simulink model "NHTSA_LDW_Straight_dashed_left_cs"  (Simulink 7.6)
settings: Solver=ode5  SolverMode=SingleTasking  StartTime=0.0  StopTime=20  FixedStep=1/100  RelTol=1e-3
PreLoadFcn:
  | check_NUTS_defined;
  | 
  | assignin('base',['model_closed_' bdroot],false);
  | 
  | if exist('LDW_mask_sfun.mexw64')==3
  | delete LDW_mask_sfun.mexw64;
  | end
  | 
  | if exist('LDW_mask_sfun.mexw32') ==3
  | delete LDW_mask_sfun.mexw32;
  | end
  | 
  | switch version('-release')
  | case {'2010a', '2010b', '2011a'}
  | addpath('../includes_LKAS/includes_LKAS_2010a');
  | case {'2011b', '2012a', '2012b'}
  | addpath('../includes_LKAS/includes_LKAS_2011b');
  | otherwise
  | addpath('../includes_LKAS/includes_LKAS_2011b');
  | end
InitFcn:
  | PreScanExperimentInitFcn(bdroot)
StopFcn:
  | PreScanExperimentStopFcn(bdroot)
undefined symbols (not defined in the file): DiscIntNeverNeededParam, InitImageOutputDir, x_ini_VRML, y_ini_VRML, z_ini_VRML
libraries: simulink x22, PreScanSimulinkLibrary x8, simulink_extras x6, dspsnks4 x2, PreScanUsefulBlocks x2, simulink_need_slupdate x1
(part 3 of 5)

== system NHTSA_LDW_Straight_dashed_left_cs/VISULightSource_Audi_A8_1/conv_FogLightFrontRight ==
  on_off : Inport
  OffColor : Constant  Value="[51   51   51  255   77   77   77  255  102  102  102  255    0    0    0  255]"
  OnColor : Constant  Value="[51   51   51  255  204  204  204  255  102  102  102  255  510  510  510  255]"
  Switch1 : Switch  Threshold=0.5
  RGBcolor : Outport
  wires:
  OffColor/1 -> Switch1/3  "off"
  OnColor/1 -> Switch1/1  "on"
  on_off/1 -> Switch1/2
  Switch1/1 -> RGBcolor/1

== system NHTSA_LDW_Straight_dashed_left_cs/VISULightSource_Audi_A8_1/conv_FogLightRearLeft ==
  on_off : Inport
  OffColor : Constant  Value="[51   51   51  255   92    0    0  255  102  102  102  255    0    0    0  255]"
  OnColor : Constant  Value="[51   51   51  255  332   51    0  255  102  102  102  255  583   10    0  255]"
  Switch1 : Switch  Threshold=0.5
  RGBcolor : Outport
  wires:
  OffColor/1 -> Switch1/3  "off"
  OnColor/1 -> Switch1/1  "on"
  on_off/1 -> Switch1/2
  Switch1/1 -> RGBcolor/1

== system NHTSA_LDW_Straight_dashed_left_cs/VISULightSource_Audi_A8_1/conv_FogLightRearRight ==
  on_off : Inport
  OffColor : Constant  Value="[51   51   51  255   92    0    0  255  102  102  102  255    0    0    0  255]"
  OnColor : Constant  Value="[51   51   51  255  332   51    0  255  102  102  102  255  583   10    0  255]"
  Switch1 : Switch  Threshold=0.5
  RGBcolor : Outport
  wires:
  OffColor/1 -> Switch1/3  "off"
  OnColor/1 -> Switch1/1  "on"
  on_off/1 -> Switch1/2
  Switch1/1 -> RGBcolor/1

== system NHTSA_LDW_Straight_dashed_left_cs/VISULightSource_Audi_A8_1/conv_IndicatorLightsLeft ==
  on_off : Inport
  OffColor : Constant  Value="[51   51   51  255  138   69    0  255  102  102  102  255    0    0    0  255]"
  OnColor : Constant  Value="[51   51   51  255  255  128    0  255  102  102  102  255  255  191    0  255]"
  Switch1 : Switch  Threshold=0.5
  RGBcolor : Outport
  wires:
  Switch1/1 -> RGBcolor/1
  on_off/1 -> Switch1/2
  OnColor/1 -> Switch1/1  "on"
  OffColor/1 -> Switch1/3  "off"

== system NHTSA_LDW_Straight_dashed_left_cs/VISULightSource_Audi_A8_1/conv_IndicatorLightsRight ==
  on_off : Inport
  OffColor : Constant  Value="[51   51   51  255  138   69    0  255  102  102  102  255    0    0    0  255]"
  OnColor : Constant  Value="[51   51   51  255  255  128    0  255  102  102  102  255  255  191    0  255]"
  Switch1 : Switch  Threshold=0.5
  RGBcolor : Outport
  wires:
  OffColor/1 -> Switch1/3  "off"
  OnColor/1 -> Switch1/1  "on"
  on_off/1 -> Switch1/2
  Switch1/1 -> RGBcolor/1

== system NHTSA_LDW_Straight_dashed_left_cs/VISULightSource_Audi_A8_1/conv_MainLightFrontLeft ==
  on_off : Inport
  OffColor : Constant  Value="[26   26   26  255   77   77   77  255  102  102  102  255    0    0    0  255]"
  OnColor : Constant  Value="[51   51   51  255  255  255  255  255  102  102  102  255  683  683  683  255]"
  Switch1 : Switch  Threshold=0.5
  RGBcolor : Outport
  wires:
  OffColor/1 -> Switch1/3  "off"
  OnColor/1 -> Switch1/1  "on"
  on_off/1 -> Switch1/2
  Switch1/1 -> RGBcolor/1

== system NHTSA_LDW_Straight_dashed_left_cs/VISULightSource_Audi_A8_1/conv_MainLightFrontRight ==
  on_off : Inport
  OffColor : Constant  Value="[26   26   26  255   77   77   77  255  102  102  102  255    0    0    0  255]"
  OnColor : Constant  Value="[51   51   51  255  255  255  255  255  102  102  102  255  683  683  683  255]"
  Switch1 : Switch  Threshold=0.5
  RGBcolor : Outport
  wires:
  OffColor/1 -> Switch1/3  "off"
  OnColor/1 -> Switch1/1  "on"
  on_off/1 -> Switch1/2
  Switch1/1 -> RGBcolor/1

== system NHTSA_LDW_Straight_dashed_left_cs/VISULightSource_Audi_A8_1/conv_MainLightRearLeft ==
  on_off : Inport
  OffColor : Constant  Value="[51   51   51  255   92    0    0  255  102  102  102  255    0    0    0  255]"
  OnColor : Constant  Value="[51   51   51  255  322   51    0  255  102  102  102  255  255   40    0  255]"
  Switch1 : Switch  Threshold=0.5
  RGBcolor : Outport
  wires:
  OffColor/1 -> Switch1/3  "off"
  OnColor/1 -> Switch1/1  "on"
  on_off/1 -> Switch1/2
  Switch1/1 -> RGBcolor/1

== system NHTSA_LDW_Straight_dashed_left_cs/VISULightSource_Audi_A8_1/conv_MainLightRearRight ==
  on_off : Inport
  OffColor : Constant  Value="[51   51   51  255   92    0    0  255  102  102  102  255    0    0    0  255]"
  OnColor : Constant  Value="[51   51   51  255  322   51    0  255  102  102  102  255  255   40    0  255]"
  Switch1 : Switch  Threshold=0.5
  RGBcolor : Outport
  wires:
  OffColor/1 -> Switch1/3  "off"
  OnColor/1 -> Switch1/1  "on"
  on_off/1 -> Switch1/2
  Switch1/1 -> RGBcolor/1

== system NHTSA_LDW_Straight_dashed_left_cs/VISULightSource_Audi_A8_1/visu_BrakeLightLeft_0 ==
  Y : Inport
  Assignment : Assignment  IndexMode=Zero-based  SampleTime=TimeStep  IndexOptions=Starting index (dialog)  Indices=PortIndex  OutputSizes=[1 1]
  Data Store Read : DataStoreRead  DataStoreName=SimCoreActuators  SampleTime=TimeStep
  Data Store Write : DataStoreWrite  DataStoreName=SimCoreActuators
  wires:
  Y/1 -> Assignment/2
  Data Store Read/1 -> Assignment/1
  Assignment/1 -> Data Store Write/1

== system NHTSA_LDW_Straight_dashed_left_cs/VISULightSource_Audi_A8_1/visu_BrakeLightRight_0 ==
  Y : Inport
  Assignment : Assignment  IndexMode=Zero-based  SampleTime=TimeStep  IndexOptions=Starting index (dialog)  Indices=PortIndex  OutputSizes=[1 1]
  Data Store Read : DataStoreRead  DataStoreName=SimCoreActuators  SampleTime=TimeStep
  Data Store Write : DataStoreWrite  DataStoreName=SimCoreActuators
  wires:
  Y/1 -> Assignment/2
  Data Store Read/1 -> Assignment/1
  Assignment/1 -> Data Store Write/1

== system NHTSA_LDW_Straight_dashed_left_cs/VISULightSource_Audi_A8_1/visu_FogLightFrontLeft_0 ==
  Y : Inport
  Assignment : Assignment  IndexMode=Zero-based  SampleTime=TimeStep  IndexOptions=Starting index (dialog)  Indices=PortIndex  OutputSizes=[1 1]
  Data Store Read : DataStoreRead  DataStoreName=SimCoreActuators  SampleTime=TimeStep
  Data Store Write : DataStoreWrite  DataStoreName=SimCoreActuators
  wires:
  Y/1 -> Assignment/2
  Data Store Read/1 -> Assignment/1
  Assignment/1 -> Data Store Write/1

== system NHTSA_LDW_Straight_dashed_left_cs/VISULightSource_Audi_A8_1/visu_FogLightFrontRight_0 ==
  Y : Inport
  Assignment : Assignment  IndexMode=Zero-based  SampleTime=TimeStep  IndexOptions=Starting index (dialog)  Indices=PortIndex  OutputSizes=[1 1]
  Data Store Read : DataStoreRead  DataStoreName=SimCoreActuators  SampleTime=TimeStep
  Data Store Write : DataStoreWrite  DataStoreName=SimCoreActuators
  wires:
  Y/1 -> Assignment/2
  Data Store Read/1 -> Assignment/1
  Assignment/1 -> Data Store Write/1

== system NHTSA_LDW_Straight_dashed_left_cs/VISULightSource_Audi_A8_1/visu_FogLightRearLeft_0 ==
  Y : Inport
  Assignment : Assignment  IndexMode=Zero-based  SampleTime=TimeStep  IndexOptions=Starting index (dialog)  Indices=PortIndex  OutputSizes=[1 1]
  Data Store Read : DataStoreRead  DataStoreName=SimCoreActuators  SampleTime=TimeStep
  Data Store Write : DataStoreWrite  DataStoreName=SimCoreActuators
  wires:
  Y/1 -> Assignment/2
  Data Store Read/1 -> Assignment/1
  Assignment/1 -> Data Store Write/1

== system NHTSA_LDW_Straight_dashed_left_cs/VISULightSource_Audi_A8_1/visu_FogLightRearRight_0 ==
  Y : Inport
  Assignment : Assignment  IndexMode=Zero-based  SampleTime=TimeStep  IndexOptions=Starting index (dialog)  Indices=PortIndex  OutputSizes=[1 1]
  Data Store Read : DataStoreRead  DataStoreName=SimCoreActuators  SampleTime=TimeStep
  Data Store Write : DataStoreWrite  DataStoreName=SimCoreActuators
  wires:
  Y/1 -> Assignment/2
  Data Store Read/1 -> Assignment/1
  Assignment/1 -> Data Store Write/1

== system NHTSA_LDW_Straight_dashed_left_cs/VISULightSource_Audi_A8_1/visu_IndicatorLightsLeft_0 ==
  Y : Inport
  Assignment : Assignment  IndexMode=Zero-based  SampleTime=TimeStep  IndexOptions=Starting index (dialog)  Indices=PortIndex  OutputSizes=[1 1]
  Data Store Read : DataStoreRead  DataStoreName=SimCoreActuators  SampleTime=TimeStep
  Data Store Write : DataStoreWrite  DataStoreName=SimCoreActuators
  wires:
  Assignment/1 -> Data Store Write/1
  Data Store Read/1 -> Assignment/1
  Y/1 -> Assignment/2

== system NHTSA_LDW_Straight_dashed_left_cs/VISULightSource_Audi_A8_1/visu_IndicatorLightsRight_0 ==
  Y : Inport
  Assignment : Assignment  IndexMode=Zero-based  SampleTime=TimeStep  IndexOptions=Starting index (dialog)  Indices=PortIndex  OutputSizes=[1 1]
  Data Store Read : DataStoreRead  DataStoreName=SimCoreActuators  SampleTime=TimeStep
  Data Store Write : DataStoreWrite  DataStoreName=SimCoreActuators
  wires:
  Y/1 -> Assignment/2
  Data Store Read/1 -> Assignment/1
  Assignment/1 -> Data Store Write/1

== system NHTSA_LDW_Straight_dashed_left_cs/VISULightSource_Audi_A8_1/visu_MainLightFrontLeft_0 ==
  Y : Inport
  Assignment : Assignment  IndexMode=Zero-based  SampleTime=TimeStep  IndexOptions=Starting index (dialog)  Indices=PortIndex  OutputSizes=[1 1]
  Data Store Read : DataStoreRead  DataStoreName=SimCoreActuators  SampleTime=TimeStep
  Data Store Write : DataStoreWrite  DataStoreName=SimCoreActuators
  wires:
  Y/1 -> Assignment/2
  Data Store Read/1 -> Assignment/1
  Assignment/1 -> Data Store Write/1

== system NHTSA_LDW_Straight_dashed_left_cs/VISULightSource_Audi_A8_1/visu_MainLightFrontRight_0 ==
  Y : Inport
  Assignment : Assignment  IndexMode=Zero-based  SampleTime=TimeStep  IndexOptions=Starting index (dialog)  Indices=PortIndex  OutputSizes=[1 1]
  Data Store Read : DataStoreRead  DataStoreName=SimCoreActuators  SampleTime=TimeStep
  Data Store Write : DataStoreWrite  DataStoreName=SimCoreActuators
  wires:
  Y/1 -> Assignment/2
  Data Store Read/1 -> Assignment/1
  Assignment/1 -> Data Store Write/1

== system NHTSA_LDW_Straight_dashed_left_cs/VISULightSource_Audi_A8_1/visu_MainLightRearLeft_0 ==
  Y : Inport
  Assignment : Assignment  IndexMode=Zero-based  SampleTime=TimeStep  IndexOptions=Starting index (dialog)  Indices=PortIndex  OutputSizes=[1 1]
  Data Store Read : DataStoreRead  DataStoreName=SimCoreActuators  SampleTime=TimeStep
  Data Store Write : DataStoreWrite  DataStoreName=SimCoreActuators
  wires:
  Y/1 -> Assignment/2
  Data Store Read/1 -> Assignment/1
  Assignment/1 -> Data Store Write/1

== system NHTSA_LDW_Straight_dashed_left_cs/VISULightSource_Audi_A8_1/visu_MainLightRearRight_0 ==
  Y : Inport
  Assignment : Assignment  IndexMode=Zero-based  SampleTime=TimeStep  IndexOptions=Starting index (dialog)  Indices=PortIndex  OutputSizes=[1 1]
  Data Store Read : DataStoreRead  DataStoreName=SimCoreActuators  SampleTime=TimeStep
  Data Store Write : DataStoreWrite  DataStoreName=SimCoreActuators
  wires:
  Y/1 -> Assignment/2
  Data Store Read/1 -> Assignment/1
  Assignment/1 -> Data Store Write/1

== system NHTSA_LDW_Straight_dashed_left_cs/VISUSteer_Audi_A8_1/conv_SteeringColumn ==
  angle [deg] : Inport
  Constant13 : Constant  Value=[0 1 0]
  Mux8 : Mux  Inputs=2
  deg2rad : Gain  Gain=pi/180
  QuaternionVisu [rad] : Outport
  wires:
  deg2rad/1 -> Mux8/2
  Constant13/1 -> Mux8/1
  Mux8/1 -> QuaternionVisu [rad]/1
  angle [deg]/1 -> deg2rad/1

== system NHTSA_LDW_Straight_dashed_left_cs/VISUSteer_Audi_A8_1/conv_SteeringWheel ==
  angle [deg] : Inport
  Constant13 : Constant  Value=[-1 0 0]
  Mux8 : Mux  Inputs=2
  deg2rad : Gain  Gain=pi/180
  QuaternionVisu [rad] : Outport
  wires:
  deg2rad/1 -> Mux8/2
  Constant13/1 -> Mux8/1
  Mux8/1 -> QuaternionVisu [rad]/1
  angle [deg]/1 -> deg2rad/1

== system NHTSA_LDW_Straight_dashed_left_cs/VISUSteer_Audi_A8_1/visu_SteeringColumn ==
  Y : Inport
  Assignment : Assignment  IndexMode=Zero-based  SampleTime=TimeStep  IndexOptions=Starting index (dialog)  Indices=PortIndex  OutputSizes=[1 1]
  Data Store Read : DataStoreRead  DataStoreName=SimCoreActuators  SampleTime=TimeStep
  Data Store Write : DataStoreWrite  DataStoreName=SimCoreActuators
  wires:
  Assignment/1 -> Data Store Write/1
  Data Store Read/1 -> Assignment/1
  Y/1 -> Assignment/2

== system NHTSA_LDW_Straight_dashed_left_cs/VISUSteer_Audi_A8_1/visu_SteeringWheel ==
  Y : Inport
  Assignment : Assignment  IndexMode=Zero-based  SampleTime=TimeStep  IndexOptions=Starting index (dialog)  Indices=PortIndex  OutputSizes=[1 1]
  Data Store Read : DataStoreRead  DataStoreName=SimCoreActuators  SampleTime=TimeStep
  Data Store Write : DataStoreWrite  DataStoreName=SimCoreActuators
  wires:
  Assignment/1 -> Data Store Write/1
  Data Store Read/1 -> Assignment/1
  Y/1 -> Assignment/2

== system NHTSA_LDW_Straight_dashed_left_cs/VISUWheels_Audi_A8_1/conv_RotWheelFL ==
  BryantISO [deg] : Inport
  Fcn10 : Fcn  Expr=cos(u(1))*sin(u(3))+sin(u(1))*sin(u(2))*cos(u(3))
  Fcn11 : Fcn  Expr=sin(u(1))*sin(u(3))-cos(u(1))*sin(u(2))*cos(u(3))
  Fcn12 : Fcn  Expr=-cos(u(2))*sin(u(3))
  Fcn13 : Fcn  Expr=cos(u(1))*cos(u(3))-sin(u(1))*sin(u(2))*sin(u(3))
  Fcn14 : Fcn  Expr=sin(u(1))*cos(u(3))+cos(u(1))*sin(u(2))*sin(u(3))
  Fcn15 : Fcn  Expr=sin(u(2))
  Fcn16 : Fcn  Expr=-sin(u(1))*cos(u(2))
  Fcn17 : Fcn  Expr=cos(u(1))*cos(u(2))
  Fcn9 : Fcn  Expr=cos(u(2))*cos(u(3))
  Mux1 : Mux  Inputs=9
  RotMat2AxisAngle : Subsystem
  deg2rad : Gain  Gain=pi/180
  xyz 2 zxy : Selector  InputPortWidth=3  IndexOptions=Index vector (dialog)  Indices=[3 1 2]  OutputSizes=1
  zxy 2 xyz : Selector  InputPortWidth=4  IndexOptions=Index vector (dialog)  Indices=[2 3 1 4]  OutputSizes=1
  QuaternionVisu [rad] : Outport
  wires:
  zxy 2 xyz/1 -> QuaternionVisu [rad]/1
  xyz 2 zxy/1 -> deg2rad/1
  deg2rad/1 -> Fcn17/1, Fcn16/1, Fcn15/1, Fcn14/1, Fcn13/1, Fcn12/1, Fcn11/1, Fcn10/1, Fcn9/1
  BryantISO [deg]/1 -> xyz 2 zxy/1  "BryantAngles rotx roty rotz Visu"
  RotMat2AxisAngle/1(Angles_Visu) -> zxy 2 xyz/1
  Mux1/1 -> RotMat2AxisAngle/1(RotMat_Visu)  "RotationMatrix Visu"
  Fcn17/1 -> Mux1/9
  Fcn16/1 -> Mux1/8
  Fcn15/1 -> Mux1/7
  Fcn14/1 -> Mux1/6
  Fcn13/1 -> Mux1/5
  Fcn12/1 -> Mux1/4
  Fcn11/1 -> Mux1/3
  Fcn10/1 -> Mux1/2
  Fcn9/1 -> Mux1/1

== system NHTSA_LDW_Straight_dashed_left_cs/VISUWheels_Audi_A8_1/conv_RotWheelFR ==
  BryantISO [deg] : Inport
  Fcn10 : Fcn  Expr=cos(u(1))*sin(u(3))+sin(u(1))*sin(u(2))*cos(u(3))
  Fcn11 : Fcn  Expr=sin(u(1))*sin(u(3))-cos(u(1))*sin(u(2))*cos(u(3))
  Fcn12 : Fcn  Expr=-cos(u(2))*sin(u(3))
  Fcn13 : Fcn  Expr=cos(u(1))*cos(u(3))-sin(u(1))*sin(u(2))*sin(u(3))
  Fcn14 : Fcn  Expr=sin(u(1))*cos(u(3))+cos(u(1))*sin(u(2))*sin(u(3))
  Fcn15 : Fcn  Expr=sin(u(2))
  Fcn16 : Fcn  Expr=-sin(u(1))*cos(u(2))
  Fcn17 : Fcn  Expr=cos(u(1))*cos(u(2))
  Fcn9 : Fcn  Expr=cos(u(2))*cos(u(3))
  Mux1 : Mux  Inputs=9
  RotMat2AxisAngle : Subsystem
  deg2rad : Gain  Gain=pi/180
  xyz 2 zxy : Selector  InputPortWidth=3  IndexOptions=Index vector (dialog)  Indices=[3 1 2]  OutputSizes=1
  zxy 2 xyz : Selector  InputPortWidth=4  IndexOptions=Index vector (dialog)  Indices=[2 3 1 4]  OutputSizes=1
  QuaternionVisu [rad] : Outport
  wires:
  zxy 2 xyz/1 -> QuaternionVisu [rad]/1
  xyz 2 zxy/1 -> deg2rad/1
  deg2rad/1 -> Fcn17/1, Fcn16/1, Fcn15/1, Fcn14/1, Fcn13/1, Fcn12/1, Fcn11/1, Fcn10/1, Fcn9/1
  BryantISO [deg]/1 -> xyz 2 zxy/1  "BryantAngles rotx roty rotz Visu"
  RotMat2AxisAngle/1(Angles_Visu) -> zxy 2 xyz/1
  Mux1/1 -> RotMat2AxisAngle/1(RotMat_Visu)  "RotationMatrix Visu"
  Fcn17/1 -> Mux1/9
  Fcn16/1 -> Mux1/8
  Fcn15/1 -> Mux1/7
  Fcn14/1 -> Mux1/6
  Fcn13/1 -> Mux1/5
  Fcn12/1 -> Mux1/4
  Fcn11/1 -> Mux1/3
  Fcn10/1 -> Mux1/2
  Fcn9/1 -> Mux1/1

== system NHTSA_LDW_Straight_dashed_left_cs/VISUWheels_Audi_A8_1/conv_RotWheelRL ==
  BryantISO [deg] : Inport
  Fcn10 : Fcn  Expr=cos(u(1))*sin(u(3))+sin(u(1))*sin(u(2))*cos(u(3))
  Fcn11 : Fcn  Expr=sin(u(1))*sin(u(3))-cos(u(1))*sin(u(2))*cos(u(3))
  Fcn12 : Fcn  Expr=-cos(u(2))*sin(u(3))
  Fcn13 : Fcn  Expr=cos(u(1))*cos(u(3))-sin(u(1))*sin(u(2))*sin(u(3))
  Fcn14 : Fcn  Expr=sin(u(1))*cos(u(3))+cos(u(1))*sin(u(2))*sin(u(3))
  Fcn15 : Fcn  Expr=sin(u(2))
  Fcn16 : Fcn  Expr=-sin(u(1))*cos(u(2))
  Fcn17 : Fcn  Expr=cos(u(1))*cos(u(2))
  Fcn9 : Fcn  Expr=cos(u(2))*cos(u(3))
  Mux1 : Mux  Inputs=9
  RotMat2AxisAngle : Subsystem
  deg2rad : Gain  Gain=pi/180
  xyz 2 zxy : Selector  InputPortWidth=3  IndexOptions=Index vector (dialog)  Indices=[3 1 2]  OutputSizes=1
  zxy 2 xyz : Selector  InputPortWidth=4  IndexOptions=Index vector (dialog)  Indices=[2 3 1 4]  OutputSizes=1
  QuaternionVisu [rad] : Outport
  wires:
  zxy 2 xyz/1 -> QuaternionVisu [rad]/1
  xyz 2 zxy/1 -> deg2rad/1
  deg2rad/1 -> Fcn17/1, Fcn16/1, Fcn15/1, Fcn14/1, Fcn13/1, Fcn12/1, Fcn11/1, Fcn10/1, Fcn9/1
  BryantISO [deg]/1 -> xyz 2 zxy/1  "BryantAngles rotx roty rotz Visu"
  RotMat2AxisAngle/1(Angles_Visu) -> zxy 2 xyz/1
  Mux1/1 -> RotMat2AxisAngle/1(RotMat_Visu)  "RotationMatrix Visu"
  Fcn17/1 -> Mux1/9
  Fcn16/1 -> Mux1/8
  Fcn15/1 -> Mux1/7
  Fcn14/1 -> Mux1/6
  Fcn13/1 -> Mux1/5
  Fcn12/1 -> Mux1/4
  Fcn11/1 -> Mux1/3
  Fcn10/1 -> Mux1/2
  Fcn9/1 -> Mux1/1

== system NHTSA_LDW_Straight_dashed_left_cs/VISUWheels_Audi_A8_1/conv_RotWheelRR ==
  BryantISO [deg] : Inport
  Fcn10 : Fcn  Expr=cos(u(1))*sin(u(3))+sin(u(1))*sin(u(2))*cos(u(3))
  Fcn11 : Fcn  Expr=sin(u(1))*sin(u(3))-cos(u(1))*sin(u(2))*cos(u(3))
  Fcn12 : Fcn  Expr=-cos(u(2))*sin(u(3))
  Fcn13 : Fcn  Expr=cos(u(1))*cos(u(3))-sin(u(1))*sin(u(2))*sin(u(3))
  Fcn14 : Fcn  Expr=sin(u(1))*cos(u(3))+cos(u(1))*sin(u(2))*sin(u(3))
  Fcn15 : Fcn  Expr=sin(u(2))
  Fcn16 : Fcn  Expr=-sin(u(1))*cos(u(2))
  Fcn17 : Fcn  Expr=cos(u(1))*cos(u(2))
  Fcn9 : Fcn  Expr=cos(u(2))*cos(u(3))
  Mux1 : Mux  Inputs=9
  RotMat2AxisAngle : Subsystem
  deg2rad : Gain  Gain=pi/180
  xyz 2 zxy : Selector  InputPortWidth=3  IndexOptions=Index vector (dialog)  Indices=[3 1 2]  OutputSizes=1
  zxy 2 xyz : Selector  InputPortWidth=4  IndexOptions=Index vector (dialog)  Indices=[2 3 1 4]  OutputSizes=1
  QuaternionVisu [rad] : Outport
  wires:
  zxy 2 xyz/1 -> QuaternionVisu [rad]/1
  xyz 2 zxy/1 -> deg2rad/1
  deg2rad/1 -> Fcn17/1, Fcn16/1, Fcn15/1, Fcn14/1, Fcn13/1, Fcn12/1, Fcn11/1, Fcn10/1, Fcn9/1
  BryantISO [deg]/1 -> xyz 2 zxy/1  "BryantAngles rotx roty rotz Visu"
  RotMat2AxisAngle/1(Angles_Visu) -> zxy 2 xyz/1
  Mux1/1 -> RotMat2AxisAngle/1(RotMat_Visu)  "RotationMatrix Visu"
  Fcn17/1 -> Mux1/9
  Fcn16/1 -> Mux1/8
  Fcn15/1 -> Mux1/7
  Fcn14/1 -> Mux1/6
  Fcn13/1 -> Mux1/5
  Fcn12/1 -> Mux1/4
  Fcn11/1 -> Mux1/3
  Fcn10/1 -> Mux1/2
  Fcn9/1 -> Mux1/1

== system NHTSA_LDW_Straight_dashed_left_cs/VISUWheels_Audi_A8_1/conv_TransWheelFL ==
  transISO [m] : Inport
  Gain1 : Gain  Gain=Gain_xISO
  Gain2 : Gain  Gain=Gain_yISO
  Gain3 : Gain  Gain=Gain_zISO
  Mux2 : Mux  Inputs=3
  Sum : Sum  Inputs=|++
  pos_ini_Visu : Subsystem
  transISO2Visu : Subsystem
  transVisu [m] : Outport
  wires:
  Gain3/1 -> Mux2/3
  Gain2/1 -> Mux2/2
  Gain1/1 -> Mux2/1
  Sum/1 -> transVisu [m]/1
  pos_ini_Visu/1(pos_ini_Visu) -> Sum/2
  Mux2/1 -> Sum/1
  transISO [m]/1 -> transISO2Visu/1(transISO)
  transISO2Visu/1(trans_x_Visu) -> Gain1/1
  transISO2Visu/2(trans_y_Visu) -> Gain2/1
  transISO2Visu/3(trans_z_Visu) -> Gain3/1

== system NHTSA_LDW_Straight_dashed_left_cs/VISUWheels_Audi_A8_1/conv_TransWheelFR ==
  transISO [m] : Inport
  Gain1 : Gain  Gain=Gain_xISO
  Gain2 : Gain  Gain=Gain_yISO
  Gain3 : Gain  Gain=Gain_zISO
  Mux2 : Mux  Inputs=3
  Sum : Sum  Inputs=|++
  pos_ini_Visu : Subsystem
  transISO2Visu : Subsystem
  transVisu [m] : Outport
  wires:
  Gain3/1 -> Mux2/3
  Gain2/1 -> Mux2/2
  Gain1/1 -> Mux2/1
  Sum/1 -> transVisu [m]/1
  pos_ini_Visu/1(pos_ini_Visu) -> Sum/2
  Mux2/1 -> Sum/1
  transISO [m]/1 -> transISO2Visu/1(transISO)
  transISO2Visu/1(trans_x_Visu) -> Gain1/1
  transISO2Visu/2(trans_y_Visu) -> Gain2/1
  transISO2Visu/3(trans_z_Visu) -> Gain3/1

== system NHTSA_LDW_Straight_dashed_left_cs/VISUWheels_Audi_A8_1/conv_TransWheelRL ==
  transISO [m] : Inport
  Gain1 : Gain  Gain=Gain_xISO
  Gain2 : Gain  Gain=Gain_yISO
  Gain3 : Gain  Gain=Gain_zISO
  Mux2 : Mux  Inputs=3
  Sum : Sum  Inputs=|++
  pos_ini_Visu : Subsystem
  transISO2Visu : Subsystem
  transVisu [m] : Outport
  wires:
  Gain3/1 -> Mux2/3
  Gain2/1 -> Mux2/2
  Gain1/1 -> Mux2/1
  Sum/1 -> transVisu [m]/1
  pos_ini_Visu/1(pos_ini_Visu) -> Sum/2
  Mux2/1 -> Sum/1
  transISO2Visu/3(trans_z_Visu) -> Gain3/1
  transISO2Visu/2(trans_y_Visu) -> Gain2/1
  transISO [m]/1 -> transISO2Visu/1(transISO)
  transISO2Visu/1(trans_x_Visu) -> Gain1/1

== system NHTSA_LDW_Straight_dashed_left_cs/VISUWheels_Audi_A8_1/conv_TransWheelRR ==
  transISO [m] : Inport
  Gain1 : Gain  Gain=Gain_xISO
  Gain2 : Gain  Gain=Gain_yISO
  Gain3 : Gain  Gain=Gain_zISO
  Mux2 : Mux  Inputs=3
  Sum : Sum  Inputs=|++
  pos_ini_Visu : Subsystem
  transISO2Visu : Subsystem
  transVisu [m] : Outport
  wires:
  Gain3/1 -> Mux2/3
  Gain2/1 -> Mux2/2
  Gain1/1 -> Mux2/1
  Sum/1 -> transVisu [m]/1
  pos_ini_Visu/1(pos_ini_Visu) -> Sum/2
  Mux2/1 -> Sum/1
  transISO2Visu/3(trans_z_Visu) -> Gain3/1
  transISO2Visu/2(trans_y_Visu) -> Gain2/1
  transISO [m]/1 -> transISO2Visu/1(transISO)
  transISO2Visu/1(trans_x_Visu) -> Gain1/1

== system NHTSA_LDW_Straight_dashed_left_cs/VISUWheels_Audi_A8_1/visu_RotWheelFL ==
  Y : Inport
  Assignment : Assignment  IndexMode=Zero-based  SampleTime=TimeStep  IndexOptions=Starting index (dialog)  Indices=PortIndex  OutputSizes=[1 1]
  Data Store Read : DataStoreRead  DataStoreName=SimCoreActuators  SampleTime=TimeStep
  Data Store Write : DataStoreWrite  DataStoreName=SimCoreActuators
  wires:
  Y/1 -> Assignment/2
  Data Store Read/1 -> Assignment/1
  Assignment/1 -> Data Store Write/1

== system NHTSA_LDW_Straight_dashed_left_cs/VISUWheels_Audi_A8_1/visu_RotWheelFR ==
  Y : Inport
  Assignment : Assignment  IndexMode=Zero-based  SampleTime=TimeStep  IndexOptions=Starting index (dialog)  Indices=PortIndex  OutputSizes=[1 1]
  Data Store Read : DataStoreRead  DataStoreName=SimCoreActuators  SampleTime=TimeStep
  Data Store Write : DataStoreWrite  DataStoreName=SimCoreActuators
  wires:
  Y/1 -> Assignment/2
  Data Store Read/1 -> Assignment/1
  Assignment/1 -> Data Store Write/1

== system NHTSA_LDW_Straight_dashed_left_cs/VISUWheels_Audi_A8_1/visu_RotWheelRL ==
  Y : Inport
  Assignment : Assignment  IndexMode=Zero-based  SampleTime=TimeStep  IndexOptions=Starting index (dialog)  Indices=PortIndex  OutputSizes=[1 1]
  Data Store Read : DataStoreRead  DataStoreName=SimCoreActuators  SampleTime=TimeStep
  Data Store Write : DataStoreWrite  DataStoreName=SimCoreActuators
  wires:
  Y/1 -> Assignment/2
  Data Store Read/1 -> Assignment/1
  Assignment/1 -> Data Store Write/1

== system NHTSA_LDW_Straight_dashed_left_cs/VISUWheels_Audi_A8_1/visu_RotWheelRR ==
  Y : Inport
  Assignment : Assignment  IndexMode=Zero-based  SampleTime=TimeStep  IndexOptions=Starting index (dialog)  Indices=PortIndex  OutputSizes=[1 1]
  Data Store Read : DataStoreRead  DataStoreName=SimCoreActuators  SampleTime=TimeStep
  Data Store Write : DataStoreWrite  DataStoreName=SimCoreActuators
  wires:
  Y/1 -> Assignment/2
  Data Store Read/1 -> Assignment/1
  Assignment/1 -> Data Store Write/1

== system NHTSA_LDW_Straight_dashed_left_cs/VISUWheels_Audi_A8_1/visu_TransWheelFL ==
  Y : Inport
  Assignment : Assignment  IndexMode=Zero-based  SampleTime=TimeStep  IndexOptions=Starting index (dialog)  Indices=PortIndex  OutputSizes=[1 1]
  Data Store Read : DataStoreRead  DataStoreName=SimCoreActuators  SampleTime=TimeStep
  Data Store Write : DataStoreWrite  DataStoreName=SimCoreActuators
  wires:
  Y/1 -> Assignment/2
  Data Store Read/1 -> Assignment/1
  Assignment/1 -> Data Store Write/1

== system NHTSA_LDW_Straight_dashed_left_cs/VISUWheels_Audi_A8_1/visu_TransWheelFR ==
  Y : Inport
  Assignment : Assignment  IndexMode=Zero-based  SampleTime=TimeStep  IndexOptions=Starting index (dialog)  Indices=PortIndex  OutputSizes=[1 1]
  Data Store Read : DataStoreRead  DataStoreName=SimCoreActuators  SampleTime=TimeStep
  Data Store Write : DataStoreWrite  DataStoreName=SimCoreActuators
  wires:
  Y/1 -> Assignment/2
  Data Store Read/1 -> Assignment/1
  Assignment/1 -> Data Store Write/1

== system NHTSA_LDW_Straight_dashed_left_cs/VISUWheels_Audi_A8_1/visu_TransWheelRL ==
  Y : Inport
  Assignment : Assignment  IndexMode=Zero-based  SampleTime=TimeStep  IndexOptions=Starting index (dialog)  Indices=PortIndex  OutputSizes=[1 1]
  Data Store Read : DataStoreRead  DataStoreName=SimCoreActuators  SampleTime=TimeStep
  Data Store Write : DataStoreWrite  DataStoreName=SimCoreActuators
  wires:
  Y/1 -> Assignment/2
  Data Store Read/1 -> Assignment/1
  Assignment/1 -> Data Store Write/1

== system NHTSA_LDW_Straight_dashed_left_cs/VISUWheels_Audi_A8_1/visu_TransWheelRR ==
  Y : Inport
  Assignment : Assignment  IndexMode=Zero-based  SampleTime=TimeStep  IndexOptions=Starting index (dialog)  Indices=PortIndex  OutputSizes=[1 1]
  Data Store Read : DataStoreRead  DataStoreName=SimCoreActuators  SampleTime=TimeStep
  Data Store Write : DataStoreWrite  DataStoreName=SimCoreActuators
  wires:
  Y/1 -> Assignment/2
  Data Store Read/1 -> Assignment/1
  Assignment/1 -> Data Store Write/1

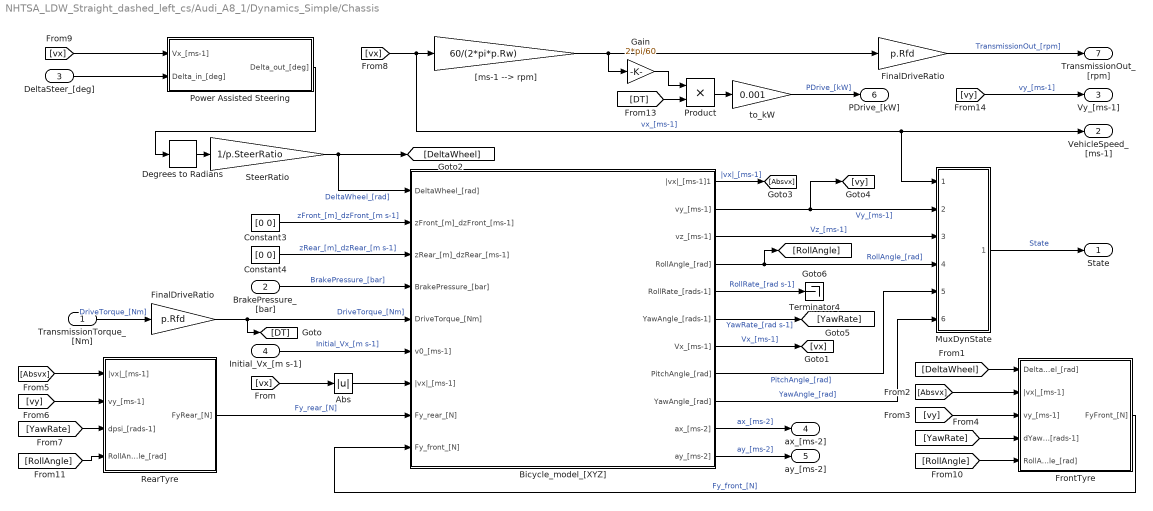
== system NHTSA_LDW_Straight_dashed_left_cs/Audi_A8_1/Dynamics_Simple/Chassis ==
  TransmissionTorque_[Nm] : Inport
  BrakePressure_[bar] : Inport  Port=2
  DeltaSteer_[deg] : Inport  Port=3
  Initial_Vx_[m s-1] : Inport  Port=4
  Abs : Abs
  Bicycle_model_[XYZ] : Subsystem
      mask Display: image(imread('Bicycle_model.png'));
  Constant3 : Constant  Value=[0 0]
  Constant4 : Constant  Value=[0 0]
  Degrees to Radians : simulink_extras/Transformations/Degrees to Radians  SystemSampleTime=-1
  FinalDriveRatio : Gain  Gain=p.Rfd  SaturateOnIntegerOverflow=on  OutDataTypeStr=Inherit: Same as input  ParamDataTypeStr=Inherit: Same as input
  "FinalDriveRatio " : Gain  Gain=p.Rfd  SaturateOnIntegerOverflow=on  OutDataTypeStr=Inherit: Same as input  ParamDataTypeStr=Inherit: Same as input
  FrontTyre : Subsystem
      mask Display: image(imread('Tyre.png'));
  Gain : Gain  Gain=2*pi/60
  MuxDynState : Subsystem
  Power Assisted Steering : Subsystem
  Product : Product  RndMeth=Zero
  RearTyre : Subsystem
      mask Display: image(imread('Tyre.png'));
  SteerRatio : Gain  Gain=1/p.SteerRatio
  Terminator4 : Terminator
  "[ms-1 --> rpm]" : Gain  Gain=60/(2*pi*p.Rw)  SaturateOnIntegerOverflow=on  OutDataTypeStr=Inherit: Same as input  ParamDataTypeStr=Inherit: Same as input
  to_kW : Gain  Gain=0.001
  State : Outport
  VehicleSpeed_[ms-1] : Outport  Port=2
  Vy_[ms-1] : Outport  Port=3
  ax_[ms-2] : Outport  Port=4
  ay_[ms-2] : Outport  Port=5
  PDrive_[kW] : Outport  Port=6
  TransmissionOut_[rpm] : Outport  Port=7
  wires:
  [vy] -> Vy_[ms-1]/1  "vy_[ms-1]"
  to_kW/1 -> PDrive_[kW]/1  "PDrive_[kW]"
  Gain/1 -> Product/1
  Bicycle_model_[XYZ]/10(ax_[ms-2]) -> ax_[ms-2]/1  "ax_[ms-2]"
  Product/1 -> to_kW/1
  [DT] -> Product/2
  Bicycle_model_[XYZ]/11(ay_[ms-2]) -> ay_[ms-2]/1  "ay_[ms-2]"
  Abs/1 -> Bicycle_model_[XYZ]/7(|vx|_[ms-1])
  Degrees to Radians/1 -> SteerRatio/1
  [vx] -> Abs/1
  SteerRatio/1 -> [DeltaWheel], Bicycle_model_[XYZ]/1(DeltaWheel_[rad])  "DeltaWheel_[rad]"
  TransmissionTorque_[Nm]/1 -> "FinalDriveRatio "/1  "DriveTorque_[Nm]"
  RearTyre/1(FyRear_[N]) -> Bicycle_model_[XYZ]/8(Fy_rear_[N])  "Fy_rear_[N]"
  FrontTyre/1(FyFront_[N]) -> Bicycle_model_[XYZ]/9(Fy_front_[N])  "Fy_front_[N]"
  Bicycle_model_[XYZ]/1(|vx|_[ms-1]1) -> [Absvx]  "|vx|_[ms-1]"
  Bicycle_model_[XYZ]/2(vy_[ms-1]) -> [vy], MuxDynState/2(vy [ms-1])  "Vy_[ms-1]"
  Bicycle_model_[XYZ]/4(RollAngle_[rad]) -> MuxDynState/4(R [rad]), [RollAngle]  "RollAngle_[rad]"
  Bicycle_model_[XYZ]/6(YawAngle_[rads-1]) -> [YawRate]  "YawRate_[rad s-1]"
  Bicycle_model_[XYZ]/7(Vx_[ms-1]) -> [vx]  "Vx_[ms-1]"
  [DeltaWheel] -> FrontTyre/1(DeltaWheel_[rad])
  [Absvx] -> FrontTyre/2(|vx|_[ms-1])
  [vy] -> FrontTyre/3(vy_[ms-1])
  [YawRate] -> FrontTyre/4(dYawAngle_[rads-1])
  [Absvx] -> RearTyre/1(|vx|_[ms-1])
  [vy] -> RearTyre/2(vy_[ms-1])
  [YawRate] -> RearTyre/3(dpsi_[rads-1])
  Bicycle_model_[XYZ]/3(vz_[ms-1]) -> MuxDynState/3(vz [ms-1])  "Vz_[ms-1]"
  Bicycle_model_[XYZ]/8(PitchAngle_[rad]) -> MuxDynState/5(P [rad])  "PitchAngle_[rad]"
  Bicycle_model_[XYZ]/9(YawAngle_[rad]) -> MuxDynState/6(Y [rad])  "YawAngle_[rad]"
  "[ms-1 --> rpm]"/1 -> Gain/1, FinalDriveRatio/1
  FinalDriveRatio/1 -> TransmissionOut_[rpm]/1  "TransmissionOut_[rpm]"
  [vx] -> "[ms-1 --> rpm]"/1, VehicleSpeed_[ms-1]/1, MuxDynState/1(vx [ms-1])  "vx_[ms-1]"
  [vx] -> Power Assisted Steering/1(Vx_[ms-1])
  DeltaSteer_[deg]/1 -> Power Assisted Steering/2(Delta_in_[deg])
  Power Assisted Steering/1(Delta_out_[deg]) -> Degrees to Radians/1
  [RollAngle] -> FrontTyre/5(RollAngle_[rad])
  [RollAngle] -> RearTyre/4(RollAngle_[rad])
  Constant3/1 -> Bicycle_model_[XYZ]/2(zFront_[m]_dzFront_[ms-1])  "zFront_[m]_dzFront_[m s-1]"
  Constant4/1 -> Bicycle_model_[XYZ]/3(zRear_[m]_dzRear_[ms-1])  "zRear_[m]_dzRear_[m s-1]"
  BrakePressure_[bar]/1 -> Bicycle_model_[XYZ]/4(BrakePressure_[bar])  "BrakePressure_[bar]"
  "FinalDriveRatio "/1 -> Bicycle_model_[XYZ]/5(DriveTorque_[Nm]), [DT]  "DriveTorque_[Nm]"
  Initial_Vx_[m s-1]/1 -> Bicycle_model_[XYZ]/6(v0_[ms-1])  "Initial_Vx_[m s-1]"
  Bicycle_model_[XYZ]/5(RollRate_[rads-1]) -> Terminator4/1  "RollRate_[rad s-1]"
  MuxDynState/1(State) -> State/1  "State"

== system NHTSA_LDW_Straight_dashed_left_cs/Audi_A8_1/Dynamics_Simple/Engine ==
  ImpellerTorque_[Nm] : Inport
  Throttle_[%] : Inport  Port=2
  Configurable Subsystem : Subsystem  BlockChoice=Discrete Rate Limiter  mask{ComputationMode=ComputationMode}
      mask prompts: ComputationMode "Compuation mode:"
      mask init:
      | SetComputationMode(gcb,ComputationMode);
      settings: AttributesFormatString=%<BlockChoice>  OpenFcn=BringToFront(gcb);  MemberBlocks=Discrete Rate Limiter,Rate Limiter
      settings: TemplateBlock=|
      | PreScanSimulinkLibrary/Configurable Subsystems/TransferFunction
      | Engine/Configurable
      | Subsystem
  Configurable Subsystem1 : Subsystem  BlockChoice=Discrete-Time Integrator  mask{ComputationMode=ComputationMode}
      mask prompts: ComputationMode "Computation mode:"
      mask init:
      | SetComputationMode(gcb,ComputationMode);
      settings: AttributesFormatString=%<BlockChoice>  OpenFcn=BringToFront(gcb);  MemberBlocks=Discrete-Time Integrator,Integrator
      settings: TemplateBlock=|
      | PreScanSimulinkLibrary/Configurable Subsystems/integral with initial condition and limts
      | for engine/Configurable
      | Subsystem
  EngineTorque : Lookup2D  RowIndex=p.thvec  ColumnIndex=p.nevec  Table=p.emap  InputSameDT=on
  Gain : Gain  Gain=2*pi/60
  Product : Product  RndMeth=Zero
  Sum : Sum  Inputs=-+  SaturateOnIntegerOverflow=on  InputSameDT=on  OutDataTypeStr=Inherit: Same as first input
  engine + impeller inertia : Gain  Gain=1/p.Iei  SaturateOnIntegerOverflow=on  OutDataTypeStr=Inherit: Same as input  ParamDataTypeStr=Inherit: Same as input
  to_kW : Gain  Gain=0.001
  nEngine_[rpm] : Outport  InitialOutput=0
  PEngine_[kW] : Outport  Port=2  InitialOutput=0
  wires:
  EngineTorque/1 -> Sum/2, Product/2
  engine + impeller inertia/1 -> Configurable Subsystem1/1(In1)
  Sum/1 -> engine + impeller inertia/1
  Configurable Subsystem1/1(Out1) -> nEngine_[rpm]/1, EngineTorque/2, Gain/1  "rpm"
  Throttle_[%]/1 -> Configurable Subsystem/1(In1)
  ImpellerTorque_[Nm]/1 -> Sum/1
  Configurable Subsystem/1(Out1) -> EngineTorque/1
  Product/1 -> to_kW/1
  Gain/1 -> Product/1
  to_kW/1 -> PEngine_[kW]/1

== system NHTSA_LDW_Straight_dashed_left_cs/Audi_A8_1/Dynamics_Simple/Gear: Auto Manual ==
  note: 0; Auto = on // Manual =off
      | 1; Auto = off // Manual =on
  Auto_Manual : Inport
  Manual_Gear : Inport  Port=2
  Auto_Gear : Inport  Port=3
  If : If  IfExpression=u1 == 0
  If Action Subsystem : Subsystem  TreatAsAtomicUnit=on
  If Action Subsystem1 : Subsystem  TreatAsAtomicUnit=on
  Merge : Merge
  Gear : Outport
  wires:
  If Action Subsystem/1(Out1) -> Merge/1
  Auto_Gear/1 -> If Action Subsystem/1(In1)
  If/1 -> If Action Subsystem/Action
  Merge/1 -> Gear/1
  If Action Subsystem1/1(Out1) -> Merge/2
  Manual_Gear/1 -> If Action Subsystem1/1(In1)
  If/2 -> If Action Subsystem1/Action
  Auto_Manual/1 -> If/1

== system NHTSA_LDW_Straight_dashed_left_cs/Audi_A8_1/Dynamics_Simple/ShiftLogic ==
  Throttle_[%] : Inport
  GearNr_[-] : Inport  Port=2
  Auto_GearShift : Inport  Port=3
  VehSpeed_[ms-1] : Inport  Port=4
  Add2 : Sum
  Data Type Conversion1 : DataTypeConversion  OutDataTypeStr=double
  Detect Increase1 : simulink/Logic and Bit Operations/Detect Increase  SystemSampleTime=-1  vinit=0.0
  Detect Increase : Subsystem
  Gear limitation : Saturate  UpperLimit=p.maxGear  LowerLimit=1
  Gear limitation while shifting : Saturate  UpperLimit=p.maxGear  LowerLimit=1
  GearNeutral : Constant  Value=0
  GearReverse : Constant  Value=-1
  "IC, gear = 1" : Memory  X0=1  InheritSampleTime=on
  If Action Neutral : Subsystem  TreatAsAtomicUnit=on
  If Action Normal : Subsystem  TreatAsAtomicUnit=on
  If Action Reverse : Subsystem  TreatAsAtomicUnit=on
  Memory : Memory  InheritSampleTime=on
  Merge : Merge  Inputs=3
  Relational Operator : RelationalOperator  OutDataTypeStr=boolean
  Relational Operator1 : RelationalOperator  Operator=<=  OutDataTypeStr=boolean
  Shift_Down time : simulink/Discrete/Integer Delay  NumDelays=p.ShiftDown_fac  InputProcessing=Inherited  vinit=0.0  samptime=-1
  Shift_Up time : simulink/Discrete/Integer Delay  NumDelays=p.ShiftUp_fac  InputProcessing=Inherited  vinit=0.0  samptime=-1
  Sum : Sum  Inputs=+-
  interp_down : Lookup2D  RowIndex=p.downth  ColumnIndex=[1:p.maxGear]  Table=p.downtab  LookUpMeth=Interpolation-Use End Values  InputSameDT=on
  interp_up : Lookup2D  RowIndex=p.upth  ColumnIndex=[1:p.maxGear]  Table=p.uptab  LookUpMeth=Interpolation-Use End Values  InputSameDT=on
  reverse/neutral/normal gear : If  IfExpression=u1 == 0  ElseIfExpressions=u1 < 0
  to_ms-1 : Gain  Gain=1/3.6
  "to_ms-1 " : Gain  Gain=1/3.6
  GearNr : Outport
  wires:
  Auto_GearShift/1 -> reverse/neutral/normal gear/1
  "IC, gear = 1"/1 -> If Action Normal/1(In1)
  Merge/1 -> GearNr/1
  If Action Reverse/1(Out1) -> Merge/2
  If Action Neutral/1(Out1) -> Merge/1
  If Action Normal/1(Out1) -> Merge/3
  reverse/neutral/normal gear/3 -> If Action Normal/Action
  reverse/neutral/normal gear/1 -> If Action Neutral/Action
  reverse/neutral/normal gear/2 -> If Action Reverse/Action
  GearReverse/1 -> If Action Reverse/1(In1)
  GearNeutral/1 -> If Action Neutral/1(In1)
  Shift_Down time/1 -> Sum/2
  Shift_Up time/1 -> Sum/1
  Detect Increase/1(Out1) -> Shift_Up time/1
  Data Type Conversion1/1 -> Shift_Down time/1
  Detect Increase1/1 -> Data Type Conversion1/1
  Sum/1 -> Add2/1
  Memory/1 -> Add2/2  "GearNr_[-]"
  Add2/1 -> Gear limitation while shifting/1
  Gear limitation while shifting/1 -> "IC, gear = 1"/1, Memory/1  "GearNr_[-]"
  Throttle_[%]/1 -> interp_down/1, interp_up/1
  Relational Operator/1 -> Detect Increase/2(In2)
  Relational Operator1/1 -> Detect Increase1/1
  interp_down/1 -> "to_ms-1 "/1
  VehSpeed_[ms-1]/1 -> Relational Operator/1, Relational Operator1/1
  interp_up/1 -> to_ms-1/1
  Gear limitation/1 -> interp_down/2, interp_up/2, Detect Increase/1(GearNr_[-])
  GearNr_[-]/1 -> Gear limitation/1
  to_ms-1/1 -> Relational Operator/2
  "to_ms-1 "/1 -> Relational Operator1/2

== system NHTSA_LDW_Straight_dashed_left_cs/Audi_A8_1/Dynamics_Simple/Transmission ==
  nEngine_[rpm] : Inport
  GearNr_[-] : Inport  Port=2
  n_TransmissionOut_[rpm] : Inport  Port=3
  Torque_Converter : Subsystem
      mask Display: image(imread('TorqueConverter.png'));
  Transmission_Ratio : Subsystem
  Viscous coupling : Lookup  InputValues=[-5:0.1:5]*p.m/4  Table=p.m/4*tanh([-5:0.1:5])
  ImpellerTorque_[Nm] : Outport  InitialOutput=0
  TransmissionTorque_[Nm] : Outport  Port=2  InitialOutput=0
  wires:
  Torque_Converter/2(TurbineTorque_[Nm]) -> Viscous coupling/1  "Converter_Torque_[Nm]"
  Transmission_Ratio/2(nTransmissionIn_[rpm]) -> Torque_Converter/2(nTransmission_[rpm])
  nEngine_[rpm]/1 -> Torque_Converter/1(nEngine_[rpm])
  GearNr_[-]/1 -> Transmission_Ratio/2(GearNr_[-]), Torque_Converter/3(Gear nr)
  n_TransmissionOut_[rpm]/1 -> Transmission_Ratio/3(nTransmissionOut_[rpm])
  Torque_Converter/1(ImpellerTorque_[Nm]) -> ImpellerTorque_[Nm]/1
  Transmission_Ratio/1(tTransmissionOut_[Nm]) -> TransmissionTorque_[Nm]/1
  Viscous coupling/1 -> Transmission_Ratio/1(tTransmissionIn_[Nm])

== system NHTSA_LDW_Straight_dashed_left_cs/Audi_A8_1/PathFollower_1/CTRL REFERENCES ==
  note: REFERENCE POSITION BASED POSITION CTRL
  Pos x,y,Y [m,m,rad] : Inport
  Position Preview Distance [m] : Inport  Port=2
  TrajOffset [m,m,rad] : Inport  Port=3
  ActorOffset_Left(+) / Right(-)_[m] : Inport  Port=4
  Calculate Preview Point (pvp) by extrapolating current Vehicle Position (p0) with Preview Distance and Vehicle Orientation : Subsystem
  Find Reference Point (pref)  on Trajectory closest  to PreView Point (pvp) : M-S-Function  FunctionName=msfcn_find_closest_trajectory_points  Parameters=[Traj_x Traj_y]
      mask Display:
      | port_label('input', 1, 'pvp')
      | port_label('input', 2, 'TrajOffset_x_y_Y')
      | port_label('input', 3, 'ActorOffset_Left+/Right-')
      | port_label('input', 4, 'p0')
      | port_label('output', 1, 'pref')
  Find Reference Point (pref0)  on Trajectory closest  to P0 Point (p0) : M-S-Function  FunctionName=msfcn_find_closest_trajectory_points0  Parameters=[Traj_x Traj_y]
      mask Display:
      | port_label('input', 1, 'pvp')
      | port_label('input', 2, 'TrajOffset_x_y_Y')
      | port_label('input', 3, 'ActorOffset_Left+/Right-')
      | port_label('input', 4, 'p0')
      | port_label('output', 1, 'pref_0')
      | port_label('output', 2, 'Actor/Traj_distance')
      | port_label('output', 3, 'Actor/Traj_angle')
  Mux1 : Mux  Inputs=2
  Selector1 : Selector  InputPortWidth=3  IndexOptions=Index vector (dialog)  Indices=[1 2]  OutputSizes=1
  Terminator : Terminator
  pvp  [m,m] : Outport
  pref_pvp [m,m] : Outport  Port=2
  pref_0 [m,m] : Outport  Port=3
  Actor/Traj_distance [m] : Outport  Port=4
  Actor/Traj_angle [deg] : Outport  Port=5
  wires:
  Mux1/1 -> pvp  [m,m]/1, Find Reference Point (pref)  on Trajectory closest  to PreView Point (pvp)/1, Find Reference Point (pref0)  on Trajectory closest  to P0 Point (p0)/1
  Pos x,y,Y [m,m,rad]/1 -> Calculate Preview Point (pvp) by extrapolating current Vehicle Position (p0) with Preview Distance and Vehicle Orientation/2(x,y,Y Demux [m,m,rad]), Find Reference Point (pref0)  on Trajectory closest  to P0 Point (p0)/4, Selector1/1
  Calculate Preview Point (pvp) by extrapolating current Vehicle Position (p0) with Preview Distance and Vehicle Orientation/1(x_glob_PVD) -> Mux1/1
  Calculate Preview Point (pvp) by extrapolating current Vehicle Position (p0) with Preview Distance and Vehicle Orientation/3(Y [rad]) -> Terminator/1
  Position Preview Distance [m]/1 -> Calculate Preview Point (pvp) by extrapolating current Vehicle Position (p0) with Preview Distance and Vehicle Orientation/1(Preview Distance)
  Find Reference Point (pref)  on Trajectory closest  to PreView Point (pvp)/1 -> pref_pvp [m,m]/1
  Find Reference Point (pref0)  on Trajectory closest  to P0 Point (p0)/1 -> pref_0 [m,m]/1
  Calculate Preview Point (pvp) by extrapolating current Vehicle Position (p0) with Preview Distance and Vehicle Orientation/2(y_glob_PVD) -> Mux1/2
  TrajOffset [m,m,rad]/1 -> Find Reference Point (pref)  on Trajectory closest  to PreView Point (pvp)/2, Find Reference Point (pref0)  on Trajectory closest  to P0 Point (p0)/2  "L6"
  ActorOffset_Left(+) / Right(-)_[m]/1 -> Find Reference Point (pref)  on Trajectory closest  to PreView Point (pvp)/3, Find Reference Point (pref0)  on Trajectory closest  to P0 Point (p0)/3
  Selector1/1 -> Find Reference Point (pref)  on Trajectory closest  to PreView Point (pvp)/4
  Find Reference Point (pref0)  on Trajectory closest  to P0 Point (p0)/2 -> Actor/Traj_distance [m]/1
  Find Reference Point (pref0)  on Trajectory closest  to P0 Point (p0)/3 -> Actor/Traj_angle [deg]/1

== system NHTSA_LDW_Straight_dashed_left_cs/Audi_A8_1/PathFollower_1/Calculate shifted p0 wrt COG ==
  position x,y,Y [m,m,deg] : Inport
  Constant1 : Constant  Value=XShifting_wrt_COG
  Degrees to Radians : simulink_extras/Transformations/Degrees to Radians  SystemSampleTime=-1
  Demux1 : Demux  Outputs=3
  Fcn : Fcn  Expr=u(2)*cos(u(1))
  Fcn1 : Fcn  Expr=u(2)*sin(u(1))
  Mux1 : Mux  Inputs=3
  Mux2 : Mux  Inputs=2
  Sum : Sum  Inputs=|++
  Sum1 : Sum  Inputs=|++
  position x,y,Y [m,m,rad] : Outport
  wires:
  Sum/1 -> Mux1/1
  Sum1/1 -> Mux1/2
  Demux1/1 -> Sum/1
  Demux1/3 -> Degrees to Radians/1
  Degrees to Radians/1 -> Mux2/1, Mux1/3
  Mux2/1 -> Fcn/1, Fcn1/1
  Fcn/1 -> Sum/2
  Fcn1/1 -> Sum1/2
  Demux1/2 -> Sum1/1
  position x,y,Y [m,m,deg]/1 -> Demux1/1
  Mux1/1 -> position x,y,Y [m,m,rad]/1
  Constant1/1 -> Mux2/2

== system NHTSA_LDW_Straight_dashed_left_cs/Audi_A8_1/PathFollower_1/DELTA CTRL ==
  note: POSITION BASED STEERWHEEL CONTROL
  p0 : Inport
  pvp : Inport  Port=2
  pref_pvp : Inport  Port=3
  pref0 : Inport  Port=4
  Calculate  preview angle : M-S-Function  FunctionName=msfcn_preview_angle_and_distance
      mask Display:
      | port_label('input', 2, 'pref [m,m]')
      | port_label('input', 3, 'p0 [m,m]')
      | port_label('input', 1, 'pvp [m,m]')
      | 
      | port_label('output', 1, 'angle [rad]')
  Divide2 : Product
  Divide4 : Product
  Error check : Subsystem
  Goto Tag Visibility : GotoTagVisibility  GotoTag=pref0
  Goto Tag Visibility1 : GotoTagVisibility  GotoTag=p0
  Radians to Degrees1 : simulink_extras/Transformations/Radians to Degrees  SystemSampleTime=-1
  Selector2 : Selector  InputPortWidth=3  IndexOptions=Index vector (dialog)  Indices=[1 2]  OutputSizes=1
  Steering angle  velocity dependent : Lookup  InputValues=[0 18 40 60 70 80 90 100 110]  Table=[16.5 16.5 28 44.5 55 60.5 60.5 60.5 60.5]
  Steering angle preview  distance dependent : Lookup  InputValues=[0 1 4 5 6 7 8 9 10 11 20 21]  Table=[1.5 1.5 1 1 1 1 1 1 0.9 0.9 0.8 0.8]
  These limits are  the vehicle maximum  steering wheel angle : Saturate  UpperLimit=720  LowerLimit=-720
  TunableSteering Gain : Gain  Gain=TunableSteeringGain
  sign1 : Gain  Gain=3.6
  delta_steerwheel [deg] : Outport
  tag scope: p0=scoped, pref0=scoped
  wires:
  Calculate  preview angle/1 -> Radians to Degrees1/1
  Selector2/1 -> Calculate  preview angle/3
  p0/1 -> Selector2/1, [p0]
  pvp/1 -> Calculate  preview angle/1
  pref_pvp/1 -> Calculate  preview angle/2
  Radians to Degrees1/1 -> Divide2/2
  These limits are  the vehicle maximum  steering wheel angle/1 -> delta_steerwheel [deg]/1
  pref0/1 -> [pref0]
  sign1/1 -> Steering angle  velocity dependent/1
  [v_actual] -> sign1/1
  Steering angle  velocity dependent/1 -> Divide2/1
  Divide4/1 -> TunableSteering Gain/1
  Divide2/1 -> Divide4/1
  Steering angle preview  distance dependent/1 -> Divide4/2
  [PreviewDistance] -> Steering angle preview  distance dependent/1
  TunableSteering Gain/1 -> These limits are  the vehicle maximum  steering wheel angle/1

== system NHTSA_LDW_Straight_dashed_left_cs/Audi_A8_1/PathFollower_1/THROTTLE CTRL ==
  v_actual [m/s] : Inport
  Desired Velocity [m/s] : Inport  Port=2
  Initial Velocity [m/s] : Inport  Port=3
  Demux : Demux  Outputs=3
  GearNormal : Constant
  "GearNormal " : Constant
  If Desired Velocity = 0 : Subsystem  TreatAsAtomicUnit=on
  If Desired Velocity ~= 0 : Subsystem  TreatAsAtomicUnit=on
  Merge : Merge
  Mux : Mux  Inputs=3
  Mux2 : Mux  Inputs=3
  Sum4 : Sum  Inputs=|+-
  if : If  IfExpression=u1 == 0
  throttle [%] : Outport
  brake pressure [bar] : Outport  Port=2
  v0 [m/s] : Outport  Port=3
  Auto_GearShift : Outport  Port=4
  wires:
  v_actual [m/s]/1 -> Sum4/2
  If Desired Velocity ~= 0/3(Auto_GearShift) -> Mux2/3
  If Desired Velocity ~= 0/2(brake pressure [bar]) -> Mux2/2
  If Desired Velocity ~= 0/1(throttle [%]) -> Mux2/1
  if/1 -> If Desired Velocity = 0/Action
  if/2 -> If Desired Velocity ~= 0/Action
  If Desired Velocity = 0/3(Auto_GearShift) -> Mux/3
  "GearNormal "/1 -> If Desired Velocity ~= 0/1(In1)
  Demux/3 -> Auto_GearShift/1
  Demux/2 -> brake pressure [bar]/1
  Demux/1 -> throttle [%]/1
  Mux/1 -> Merge/1
  Mux2/1 -> Merge/2
  If Desired Velocity = 0/2(brake pressure [bar]) -> Mux/2
  If Desired Velocity = 0/1(throttle [%]) -> Mux/1
  Merge/1 -> Demux/1
  GearNormal/1 -> If Desired Velocity = 0/1(In1)
  Initial Velocity [m/s]/1 -> v0 [m/s]/1
  Desired Velocity [m/s]/1 -> Sum4/1, if/1
  Sum4/1 -> If Desired Velocity ~= 0/2(Desired Velocity [m/s])

== system NHTSA_LDW_Straight_dashed_left_cs/Audi_A8_1/SELF_Demux/compas converter ==
  rotz [rad] : Inport
  cart2compas : Subsystem
  rad2deg : Gain  Gain=180/pi
  heading [deg] : Outport
  wires:
  cart2compas/1(heading [deg]) -> heading [deg]/1
  rotz [rad]/1 -> rad2deg/1
  rad2deg/1 -> cart2compas/1(Angle [deg])
